simulink model "W04_P1"  (R2024b)
settings: Solver=ode4  StartTime=0  StopTime=T_final  FixedStep=h  RelTol=1e-3
values from neighbouring files (symbols this model uses):
  x0 = zeros(12,1);  x0(12) = deg2rad(170)    [W04_check.m]
undefined symbols (not defined in the file or in its folder): beta_c, k_neg, k_pos, mp, n_max, n_min, rp, V_c, X_ff, y_pont
settings Model: Creator=admin  LastModifiedBy=admin
settings DataIOCC: ReturnWorkspaceOutputs=off

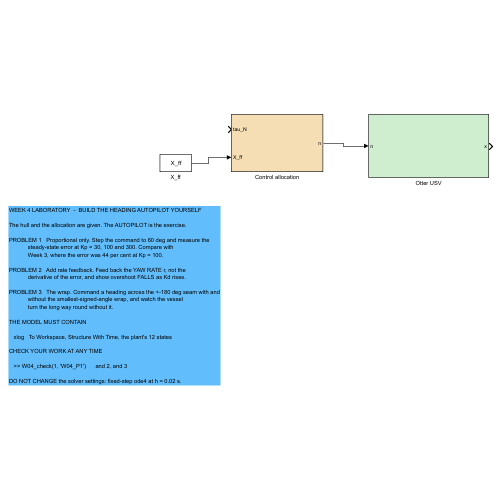
[thumbnail: Simulink's stored preview of the top-level diagram]
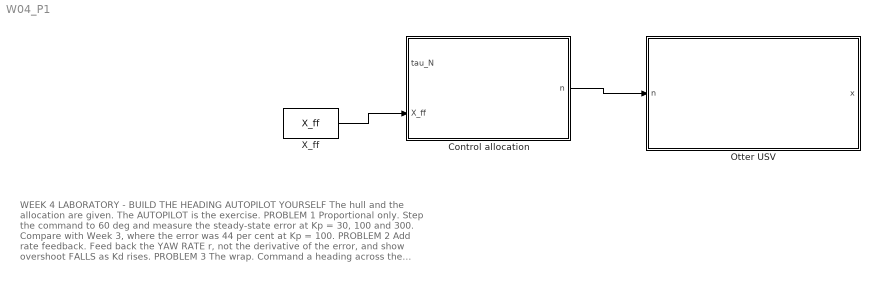
== system W04_P1 ==
  note: WEEK 4 LABORATORY  -  BUILD THE HEADING AUTOPILOT YOURSELF
      |
      | The hull and the allocation are given. The AUTOPILOT is the exercise.
      |
      | PROBLEM 1   Proportional only. Step the command to 60 deg and measure the
      |             steady-state error at Kp = 30, 100 and 300. Compare with
      |             Week 3, where the error was 44 per cent at Kp = 100.
      |
      | PROBLEM 2   Add rate feedback. Feed back the YAW RATE r, not the
      |             derivative of the error, and show overshoot FALLS as Kd rises.
      |
      | PROBLEM 3   The wrap. Command a heading across the +-180 deg seam with and
      |             without the smallest-signed-angle wrap, and watch the vessel
      |             turn the long way round without it.
      |
      | THE MODEL MUST CONTAIN
      |
      |    xlog   To Workspace, Structure With Time, the plant's 12 states
      |
      | CHECK YOUR WORK AT ANY TIME
      |
      |    >> W04_check(1, 'W04_P1')      and 2, and 3
      |
      | DO NOT CHANGE the solver settings: fixed-step ode4 at h = 0.02 s.
  Control allocation : Subsystem
  Otter USV : Subsystem
  X_ff : Constant  Value=X_ff
  wires:
  Control allocation/1(n) -> Otter USV/1(n)
  X_ff/1 -> Control allocation/2(X_ff)

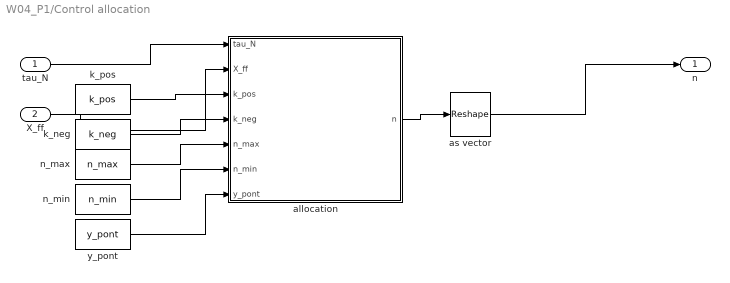
== system W04_P1/Control allocation ==
  tau_N : Inport
  X_ff : Inport  Port=2
  allocation : MATLAB Function  TreatAsAtomicUnit=on
  as vector : Reshape
  k_neg : Constant  Value=k_neg
  k_pos : Constant  Value=k_pos
  n_max : Constant  Value=n_max
  n_min : Constant  Value=n_min
  y_pont : Constant  Value=y_pont
  n : Outport
  wires:
  k_pos/1 -> allocation/3(k_pos)
  k_neg/1 -> allocation/4(k_neg)
  n_max/1 -> allocation/5(n_max)
  n_min/1 -> allocation/6(n_min)
  y_pont/1 -> allocation/7(y_pont)
  tau_N/1 -> allocation/1(tau_N)
  X_ff/1 -> allocation/2(X_ff)
  allocation/1(n) -> as vector/1
  as vector/1 -> n/1

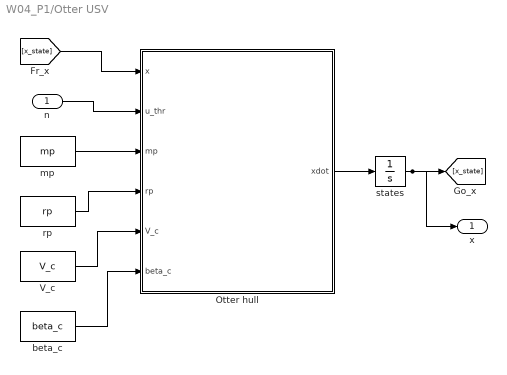
== system W04_P1/Otter USV ==
  n : Inport
  Otter hull : MATLAB Function  TreatAsAtomicUnit=on
  V_c : Constant  Value=V_c
  beta_c : Constant  Value=beta_c
  mp : Constant  Value=mp
  rp : Constant  Value=rp
  states : Integrator  InitialCondition=x0
  x : Outport
  wires:
  [x_state] -> Otter hull/1(x)
  n/1 -> Otter hull/2(u_thr)
  mp/1 -> Otter hull/3(mp)
  Otter hull/1(xdot) -> states/1
  beta_c/1 -> Otter hull/6(beta_c)
  rp/1 -> Otter hull/4(rp)
  states/1 -> [x_state], x/1
  V_c/1 -> Otter hull/5(V_c)

== matlab function W04_P1/Otter USV/Otter hull ==
  data: x input; xdot output double size=[12 1]; u_thr input; mp input; rp input; V_c input; beta_c input
function xdot = otter_hull(x, u_thr, mp, rp, V_c, beta_c)
% Fossen's otter.m, called unchanged from Tools/MSS/VESSELS.
%
%   x       12 states, fed back from the integrator
%   u_thr   propeller shaft speeds [rad/s]
%
% otter.m is not written for code generation, so the call is extrinsic and
% xdot has to be pre-sized for Simulink to know the output width.
coder.extrinsic('otter');

xdot = zeros(12,1);
xdot = otter(x, u_thr, mp, rp, V_c, beta_c);
end

== matlab function W04_P1/Control allocation/allocation ==
  data: tau_N input; n output double size=[2 1]; X_ff input; k_pos input; k_neg input; n_max input; n_min input; y_pont input
function n = allocation(tau_N, X_ff, k_pos, k_neg, n_max, n_min, y_pont)
%#codegen
% Demanded surge force and yaw moment to two shaft speeds.
%
% Step 1, the exact inverse of tau = B f:
%     T1 = X/2 + N/(2 y_pont)
%     T2 = X/2 - N/(2 y_pont)
%
% Step 2, the propeller curve inverted one propeller at a time:
%     n = sign(T) sqrt(|T| / k),  with k_pos ahead and k_neg astern.
T = [X_ff/2 + tau_N/(2*y_pont);
     X_ff/2 - tau_N/(2*y_pont)];
n = zeros(2,1);
for i = 1:2
    if T(i) >= 0
        ni =  sqrt( T(i) / k_pos);
    else
        ni = -sqrt(-T(i) / k_neg);
    end
    n(i) = min(max(ni, n_min), n_max);
end
end
